simulink model "CA_4"  (R2021b)
settings: Solver=ode45  StartTime=0.0  StopTime=100  MaxStep=1e-3  RelTol=1e-3
settings Model: Creator=Farbod  LastModifiedBy=hp
settings SolverCC: AlgebraicLoopSolver=TrustRegion
settings DataIOCC: ReturnWorkspaceOutputs=off
settings OptimizationCC: LifeSpan=inf
settings DebuggingCC: SFExecutionAtInitializationDiag=none  SFMachineParentedDataDiag=warning  ArithmeticOperatorsInVariantConditions=warning
settings HardwareCC: ProdBitPerSizeT=32  ProdBitPerPtrDiffT=32  ProdWordSize=32  ProdHWDeviceType=Specified
settings SFSimCC: SimUseLocalCustomCode=off  CustomCodeUndefinedFunction=UseInterfaceOnly
settings RTWCC: RTWUseLocalCustomCode=off
settings CodeAppCC: StateflowObjectComments=on

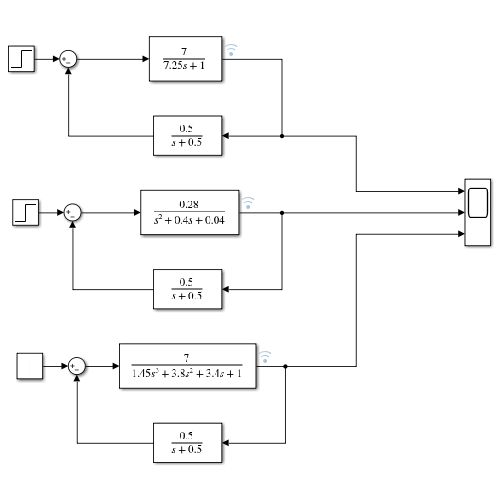
[thumbnail: Simulink's stored preview of the top-level diagram]
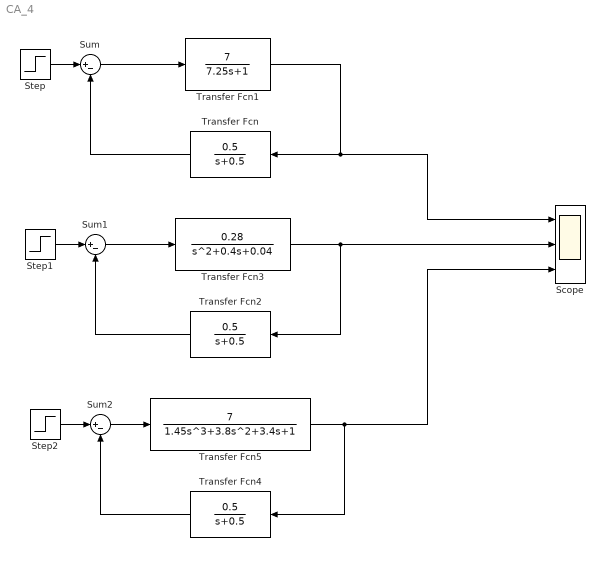
== system CA_4 ==
  Scope : Scope  NumInputPorts=3
  Step : Step  SampleTime=0
  Step1 : Step  SampleTime=0
  Step2 : Step  SampleTime=0
  Sum : Sum  Inputs=|+-
  Sum1 : Sum  Inputs=|+-
  Sum2 : Sum  Inputs=|+-
  Transfer Fcn : TransferFcn  Numerator=[0.5]  Denominator=[1 0.5]
  Transfer Fcn1 : TransferFcn  Numerator=[7]  Denominator=[7.25 1]
  Transfer Fcn2 : TransferFcn  Numerator=[0.5]  Denominator=[1 0.5]
  Transfer Fcn3 : TransferFcn  Numerator=[0.28]  Denominator=[1 0.4 0.04]
  Transfer Fcn4 : TransferFcn  Numerator=[0.5]  Denominator=[1 0.5]
  Transfer Fcn5 : TransferFcn  Numerator=[7]  Denominator=[1.45 3.8 3.4 1]
  wires:
  Transfer Fcn/1 -> Sum/2
  Transfer Fcn1/1 -> Transfer Fcn/1, Scope/1
  Sum/1 -> Transfer Fcn1/1
  Step/1 -> Sum/1
  Sum1/1 -> Transfer Fcn3/1
  Transfer Fcn2/1 -> Sum1/2
  Step1/1 -> Sum1/1
  Sum2/1 -> Transfer Fcn5/1
  Step2/1 -> Sum2/1
  Transfer Fcn3/1 -> Transfer Fcn2/1, Scope/2
  Transfer Fcn5/1 -> Transfer Fcn4/1, Scope/3
  Transfer Fcn4/1 -> Sum2/2
